simulink subsystem "Subsystem_Controlador_ACT"  (R2023b)
settings: Solver=VariableStepAuto  StartTime=0.0  StopTime=10.0  RelTol=1e-3
settings Model: Creator=Alberto  LastModifiedBy=Alberto

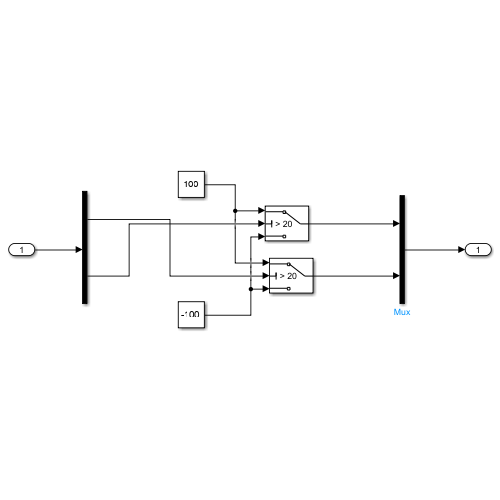
[thumbnail: Simulink's stored preview of the top-level diagram]
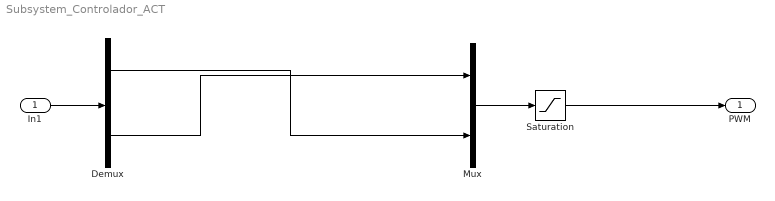
== system Subsystem_Controlador_ACT ==
  In1 : Inport
  Demux : Demux  Outputs=2
  Mux : Mux  Inputs=2
  Saturation : Saturate  UpperLimit=100  LowerLimit=0
  PWM : Outport
  wires:
  Mux/1 -> Saturation/1
  In1/1 -> Demux/1
  Demux/1 -> Mux/2
  Demux/2 -> Mux/1
  Saturation/1 -> PWM/1
